simulink model "Dynamic_Modelspeed"  (R2023a)
settings: Solver=ode4  StartTime=0.0  StopTime=1.5  FixedStep=Ts  RelTol=1e-3
InitFcn:
  | eval  SRM_Parameters ;
undefined symbols (not defined in the file): B, Curr_F_4Q_MH, di, DiscIntNeverNeededParam, I_peak, J, KD, KI, KP, sigbuilder_block, T_4Q_MH, Ts, Vdc
libraries: simulink x3, dspsigops x1
(part 1 of 5)
settings Model: Creator=Fahad  LastModifiedBy=user
settings SolverCC: AlgebraicLoopSolver=LineSearch
settings DataIOCC: ReturnWorkspaceOutputs=off
settings OptimizationCC: ReuseModelBlockBuffer=off  LifeSpan=inf
settings DebuggingCC: UnconnectedInputMsg=warning  UnconnectedOutputMsg=warning  UnconnectedLineMsg=warning  SFExecutionAtInitializationDiag=none  ArithmeticOperatorsInVariantConditions=warning
settings ModelReferenceCC: EnableRefExpFcnMdlSchedulingChecks=on
settings SFSimCC: SimUseLocalCustomCode=off  CustomCodeUndefinedFunction=UseInterfaceOnly
settings RTWCC: RTWUseLocalCustomCode=off  DLArmComputeVersion=19.05
settings CodeAppCC: StateflowObjectComments=on

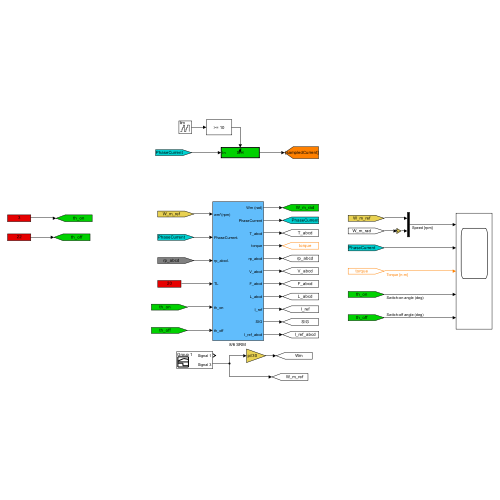
[thumbnail: Simulink's stored preview of the top-level diagram]
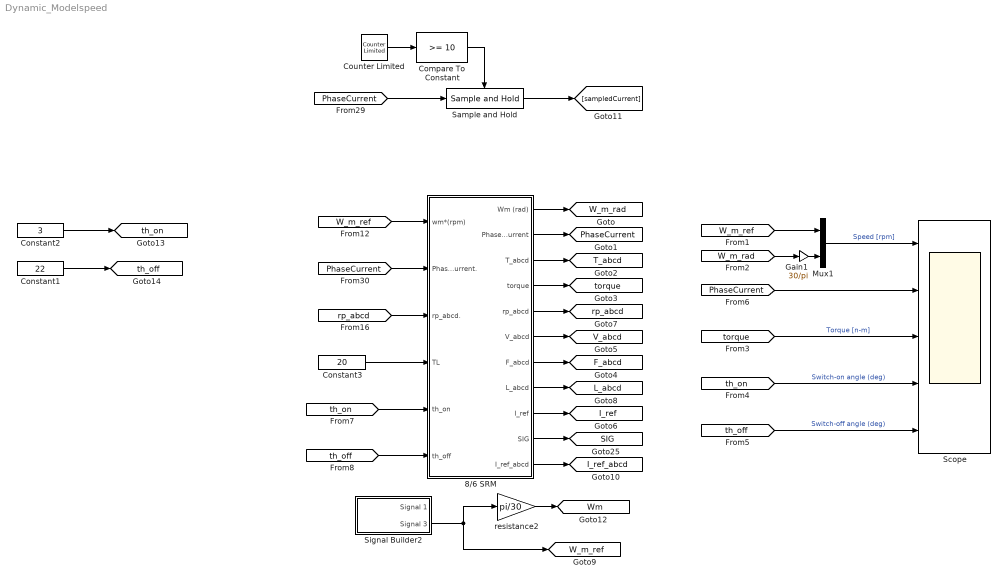
== system Dynamic_Modelspeed ==
  "8/6 SRM " : Subsystem
  Compare To Constant : simulink/Logic and Bit Operations/Compare To Constant  relop=>=  const=10  OutDataTypeStr=boolean
  Constant1 : Constant  Value=22
  Constant2 : Constant  Value=3
  Constant3 : Constant  Value=20
  Counter Limited : simulink/Sources/Counter Limited  uplimit=10  tsamp=Ts
  Gain1 : Gain  Gain=30/pi
  Mux1 : Mux  Inputs=2
  Sample and Hold : dspsigops/Sample and Hold  trig=Rising edge  initCond=0  latchinput=off
  Scope : Scope  NumInputPorts=5
  Signal Builder2 : Subsystem  Tag=STV Subsys  LoadFcn=sigbuilder_block('load');  StartFcn=sigbuilder_block('start');  StopFcn=sigbuilder_block('stop');  ClipboardFcn=sigbuilder_block('clipboard');  mask(Sigbuilder block){tuvar=[0:10]}
      mask help: Simulink:masks:SigbuilderBlock_MD
      mask init:
      | if ~strcmp(get_param(bdroot(gcbh),'SimulationStatus'),'stopped') tuvar = sigbuilder_block('maskInit'); end
      settings: CopyFcn=sigbuilder_block('copy');  DeleteFcn=sigbuilder_block('delete');  ModelCloseFcn=sigbuilder_block('modelClose');  PreSaveFcn=sigbuilder_block('preSave');  PauseFcn=sigbuilder_block('pause');  ContinueFcn=sigbuilder_block('continue');  NameChangeFcn=sigbuilder_block('namechange');  OpenFcn=sigbuilder_block('open',[236.4 90.6 550.8 361.2 ]);  CloseFcn=sigbuilder_block('close');
      mask Display: plot(0, 0, 100, 100,[2, 2, 32, 32, 2], [68, 8, 8, 68, 68],[32, 2], [38, 38], [32, 19, 2],[53, 60, 44], [32, 17, 17, 2],[16, 16, 31, 31]);txt = getActiveGroup(gcbh);text(2, 100, txt,'verticalAlignment', 'top');
  resistance2 : Gain  Gain=pi/30
  tag scope: F_abcd=global, I_ref=global, I_ref_abcd=global, L_abcd=global, PhaseCurrent=global, SIG=global, T_abcd=global, V_abcd=global, W_m_rad=global, W_m_ref=global, Wm=global, rp_abcd=global, th_off=global, th_on=global, torque=global
  wires:
  "8/6 SRM "/9(I_ref) -> [I_ref]
  "8/6 SRM "/4(torque) -> [torque]
  [PhaseCurrent] -> "8/6 SRM "/2(PhaseCurrent.)
  "8/6 SRM "/3(T_abcd) -> [T_abcd]
  "8/6 SRM "/10(SIG) -> [SIG]
  "8/6 SRM "/7(F_abcd) -> [F_abcd]
  "8/6 SRM "/2(PhaseCurrent) -> [PhaseCurrent]
  "8/6 SRM "/8(L_abcd) -> [L_abcd]
  "8/6 SRM "/6(V_abcd) -> [V_abcd]
  [W_m_ref] -> "8/6 SRM "/1(wm*(rpm))
  "8/6 SRM "/1(Wm (rad)) -> [W_m_rad]
  "8/6 SRM "/5(rp_abcd) -> [rp_abcd]
  [rp_abcd] -> "8/6 SRM "/3(rp_abcd.)
  "8/6 SRM "/11(I_ref_abcd) -> [I_ref_abcd]
  resistance2/1 -> [Wm]
  [PhaseCurrent] -> Sample and Hold/1
  Sample and Hold/1 -> [sampledCurrent]
  Compare To Constant/1 -> Sample and Hold/Trigger
  Counter Limited/1 -> Compare To Constant/1
  Constant3/1 -> "8/6 SRM "/4(TL)
  [th_off] -> Scope/5  "Switch-off angle (deg)"
  [torque] -> Scope/3  "Torque [n-m]"
  Gain1/1 -> Mux1/2
  [th_on] -> Scope/4  "Switch-on angle (deg)"
  [W_m_rad] -> Gain1/1
  [W_m_ref] -> Mux1/1
  [th_off] -> "8/6 SRM "/6(th_off)
  Mux1/1 -> Scope/1  "Speed [rpm]"
  [PhaseCurrent] -> Scope/2
  Constant1/1 -> [th_off]
  Constant2/1 -> [th_on]
  [th_on] -> "8/6 SRM "/5(th_on)
  Signal Builder2/2(Signal 3) -> resistance2/1, [W_m_ref]

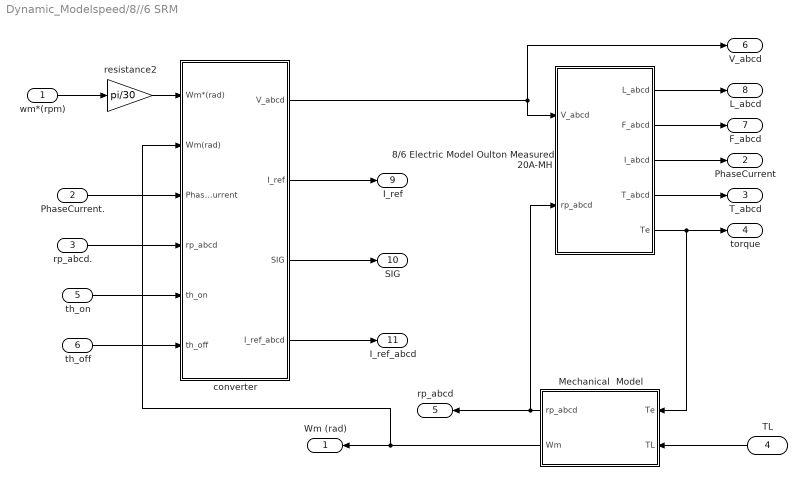
== system Dynamic_Modelspeed/8//6 SRM  ==
  wm*(rpm) : Inport
  PhaseCurrent. : Inport  Port=2
  rp_abcd. : Inport  Port=3
  TL : Inport  Port=4
  th_on : Inport  Port=5
  th_off : Inport  Port=6
  8/6 Electric Model Oulton Measured 20A-MH : Subsystem
  Mechanical  Model : Subsystem
  converter : Subsystem
  resistance2 : Gain  Gain=pi/30
  Wm (rad) : Outport
  PhaseCurrent : Outport  Port=2
  T_abcd : Outport  Port=3
  torque : Outport  Port=4
  rp_abcd : Outport  Port=5
  V_abcd : Outport  Port=6
  F_abcd : Outport  Port=7
  L_abcd : Outport  Port=8
  I_ref : Outport  Port=9
  SIG : Outport  Port=10
  I_ref_abcd : Outport  Port=11
  wires:
  converter/1(V_abcd) -> 8/6 Electric Model Oulton Measured 20A-MH/1(V_abcd), V_abcd/1
  8/6 Electric Model Oulton Measured 20A-MH/4(T_abcd) -> T_abcd/1
  8/6 Electric Model Oulton Measured 20A-MH/3(I_abcd) -> PhaseCurrent/1
  8/6 Electric Model Oulton Measured 20A-MH/2(F_abcd) -> F_abcd/1
  8/6 Electric Model Oulton Measured 20A-MH/1(L_abcd) -> L_abcd/1
  8/6 Electric Model Oulton Measured 20A-MH/5(Te) -> Mechanical  Model/1(Te), torque/1
  PhaseCurrent./1 -> converter/3(PhaseCurrent)
  TL/1 -> Mechanical  Model/2(TL)
  Mechanical  Model/1(rp_abcd) -> 8/6 Electric Model Oulton Measured 20A-MH/2(rp_abcd), rp_abcd/1
  converter/3(SIG) -> SIG/1
  converter/2(I_ref) -> I_ref/1
  rp_abcd./1 -> converter/4(rp_abcd)
  wm*(rpm)/1 -> resistance2/1
  resistance2/1 -> converter/1(Wm*(rad))
  Mechanical  Model/2(Wm) -> converter/2(Wm(rad)), Wm (rad)/1
  converter/4(I_ref_abcd) -> I_ref_abcd/1
  th_off/1 -> converter/6(th_off)
  th_on/1 -> converter/5(th_on)

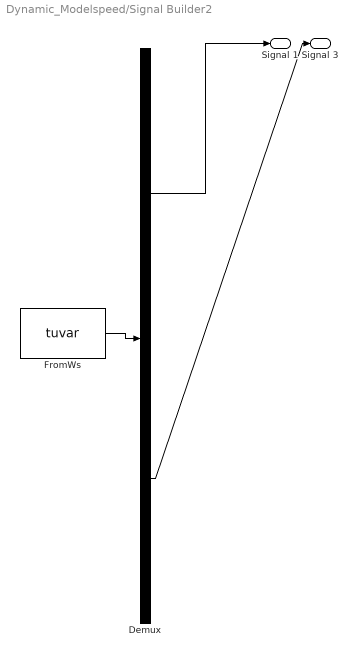
== system Dynamic_Modelspeed/Signal Builder2 ==
  Demux : Demux  Tag=STV Demux  Outputs=2
      settings: DisplayOption=none
  FromWs : FromWorkspace  Tag=STV FromWs  VariableName=tuvar
      SigBuilderData=|
      | common.afterFinalStr = 'Extrapolate'
      | common.sampleTime = 0
      | dataSet.timeRange = [0 1.5]
      | dataSet.name = 'Group 1'
      | sbobj.Groups.Name = 'Group 1'
      | sbobj.Groups.Signals(1).Name = 'Signal 1'
      | sbobj.Groups.Signals(1).XData = [0 0.5 0.5 1 1 1.5]
      | sbobj.Groups.Signals(1).YData = [300 300 1000 1000 2000 2000]
      | sbobj.Groups.Signals(2).Name = 'Signal 3'
      | sbobj.Groups.Signals(2).XData = [0 0.27 0.27 0.7 0.7 1.5]
      | sbobj.Groups.Signals(2).YData = [300 300 900 900 1500 1500]
      | sbobj.Groups.TimeRange = [0 1.5]
  Signal 1 : Outport  Tag=STV Outport
  Signal 3 : Outport  Tag=STV Outport  Port=2
  wires:
  Demux/1 -> Signal 1/1
  FromWs/1 -> Demux/1
  Demux/2 -> Signal 3/1
